simulink model "FSAE_UnifiedControl_ClosedLoop"  (R2026a)
settings: Solver=ode45  StopTime=10  MaxStep=0.01
model workspace (MAT data in the model file):
  PathTrackingAntiWindupGain = 0.5
  PathTrackingBrakePressurePerAcceleration = 10000
  PathTrackingControlSampleTime = 0.01
  PathTrackingCrossTrackGain = 2
  PathTrackingEnvironment.RoadGripScale = [1; 1; 1; 1]
  PathTrackingEnvironment.RoadMuLimit = [Inf; Inf; Inf; Inf]
  PathTrackingEnvironment.RoadGrade = 0
  PathTrackingEnvironment.RoadBank = 0
  PathTrackingEnvironment.RoadHeight = [0; 0; 0; 0]
  PathTrackingEnvironment.AirDensity = 1.225
  PathTrackingEnvironment.WindVelocityGlobal = [0; 0; 0]
  PathTrackingEnvironment.AmbientTemperature = 25
  PathTrackingEnvironment.Gravity = 9.80665
  PathTrackingEnvironment.EnableRoadDisturbance = 0
  PathTrackingEnvironment.EnvironmentValid = 1
  PathTrackingHeadingGain = 1.2
  PathTrackingLookaheadTime = 0.1
  PathTrackingMaximumAcceleration = 8
  PathTrackingMaximumDeceleration = 8
  PathTrackingMaximumSteeringAngle = 0.5
  PathTrackingMaximumSteeringRate = 4
  PathTrackingMinLookahead = 0.5
  PathTrackingMinimumSteeringSpeed = 1
  PathTrackingProjectionSearchWindow = 200
  PathTrackingSpeedKi = 0.25
  PathTrackingSpeedKp = 0.8
  PathTrackingSteeringWheelRatio = 1
  PathTrackingTrackData.SampleCount = 150
  PathTrackingTrackData.SampleDistance = 0.503355704698
  PathTrackingTrackData.TrackLength = 75
  PathTrackingTrackData.IsClosed = 0
  PathTrackingTrackData.ReferencePathValid = 0
  PathTrackingTrackData.ReferenceSampleDistance = 0.503355704698
  PathTrackingTrackData.X = [0 0.503355704698 1.0067114094 1.51006711409 2.01342281879 2.51677852349 3.02013422819 3.52348993289 4.02684563758 4.53020134228 5.03355704698 5.53691275168 ... (4096 elements, 4096x1)]
  PathTrackingTrackData.Y = [0 0 0 0 0 0 0 0 0 0 0 0 ... (4096 elements, 4096x1)]
  PathTrackingTrackData.Heading = [0 0 0 0 0 0 0 0 0 0 0 0 ... (4096 elements, 4096x1)]
  PathTrackingTrackData.Curvature = [0 0 0 0 0 0 0 0 0 0 0 0 ... (4096 elements, 4096x1)]
  PathTrackingTrackData.ReferenceX = [0 0.503355704698 1.0067114094 1.51006711409 2.01342281879 2.51677852349 3.02013422819 3.52348993289 4.02684563758 4.53020134228 5.03355704698 5.53691275168 ... (4096 elements, 4096x1)]
  PathTrackingTrackData.ReferenceY = [0 0 0 0 0 0 0 0 0 0 0 0 ... (4096 elements, 4096x1)]
  PathTrackingTrackData.ReferenceHeading = [0 0 0 0 0 0 0 0 0 0 0 0 ... (4096 elements, 4096x1)]
  PathTrackingTrackData.ReferenceCurvature = [0 0 0 0 0 0 0 0 0 0 0 0 ... (4096 elements, 4096x1)]
  PathTrackingTrackData.ReferenceEnvelopeClearance = [1.79769313486e+308 1.79769313486e+308 1.79769313486e+308 1.79769313486e+308 1.79769313486e+308 1.79769313486e+308 1.79769313486e+308 1.79769313486e+308 1.79769313486e+308 1.79769313486e+308 1.79769313486e+308 1.79769313486e+308 ... (4096 elements, 4096x1)]
  PathTrackingTrackData.ReferenceBoundaryCorrectionSign = [0 0 0 0 0 0 0 0 0 0 0 0 ... (4096 elements, 4096x1)]
  PathTrackingTrackData.ReferenceSpeed = [30 30 30 30 30 30 30 30 30 30 30 30 ... (4096 elements, 4096x1)]
  PathTrackingTrackData.LeftHalfWidth = [1.5 1.5 1.5 1.5 1.5 1.5 1.5 1.5 1.5 1.5 1.5 1.5 ... (4096 elements, 4096x1)]
  PathTrackingTrackData.RightHalfWidth = [1.5 1.5 1.5 1.5 1.5 1.5 1.5 1.5 1.5 1.5 1.5 1.5 ... (4096 elements, 4096x1)]
  PathTrackingWheelbase = 2
undefined symbols (not defined in the file): DefaultPowertrainStateBus, DefaultSensorBus
settings Model: DataDictionary=VehicleData.sldd  Creator=Xu Dingyi  LastModifiedBy=Xu Dingyi
settings SolverCC: ZeroCrossAlgorithm=Adaptive
settings DebuggingCC: AlgebraicLoopMsg=error  IgnoredZcDiagnostic=none  BusObjectLabelMismatch=error

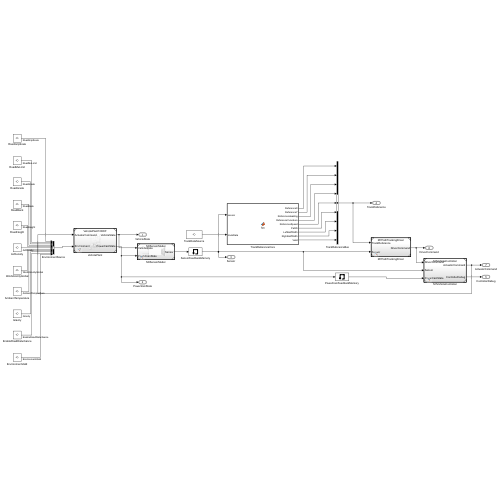
[thumbnail: Simulink's stored preview of the top-level diagram]
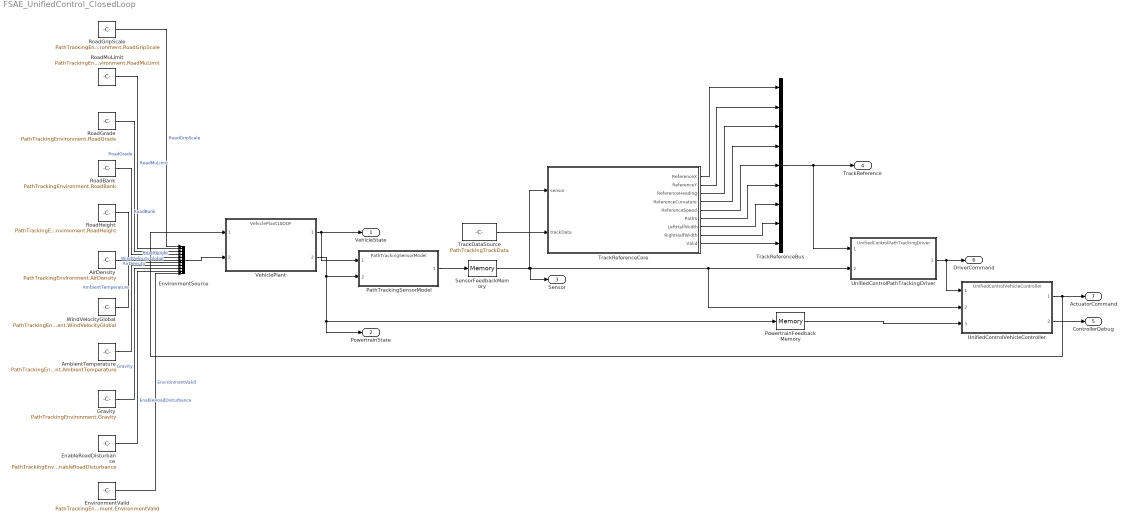
== system FSAE_UnifiedControl_ClosedLoop ==
  AirDensity : Constant  Value=PathTrackingEnvironment.AirDensity
  AmbientTemperature : Constant  Value=PathTrackingEnvironment.AmbientTemperature
  EnableRoadDisturbance : Constant  Value=PathTrackingEnvironment.EnableRoadDisturbance
  EnvironmentSource : BusCreator  Inputs=11  OutDataTypeStr=Bus: EnvironmentBus
  EnvironmentValid : Constant  Value=PathTrackingEnvironment.EnvironmentValid
  Gravity : Constant  Value=PathTrackingEnvironment.Gravity
  PathTrackingSensorModel : ModelReference  ModelNameDialog=PathTrackingSensorModel  SimulationMode=Normal  ModelReferenceVersion=1.2
  PowertrainFeedbackMemory : Memory  InitialCondition=DefaultPowertrainStateBus
  RoadBank : Constant  Value=PathTrackingEnvironment.RoadBank
  RoadGrade : Constant  Value=PathTrackingEnvironment.RoadGrade
  RoadGripScale : Constant  Value=PathTrackingEnvironment.RoadGripScale
  RoadHeight : Constant  Value=PathTrackingEnvironment.RoadHeight
  RoadMuLimit : Constant  Value=PathTrackingEnvironment.RoadMuLimit
  SensorFeedbackMemory : Memory  InitialCondition=DefaultSensorBus
  TrackDataSource : Constant  Value=PathTrackingTrackData  OutDataTypeStr=Bus: PathTrackingTrackDataBus
  TrackReferenceBus : BusCreator  Inputs=9  OutDataTypeStr=Bus: TrackReferenceBus
  TrackReferenceCore : MATLAB Function  TreatAsAtomicUnit=on
  UnifiedControlPathTrackingDriver : ModelReference  ModelNameDialog=UnifiedControlPathTrackingDriver  SimulationMode=Normal  ModelReferenceVersion=1.2
  UnifiedControlVehicleController : ModelReference  ModelNameDialog=UnifiedControlVehicleController  SimulationMode=Normal  ModelReferenceVersion=1.2
  VehiclePlant : ModelReference  ModelNameDialog=VehiclePlant10DOF  SimulationMode=Normal  ModelReferenceVersion=1.22
  WindVelocityGlobal : Constant  Value=PathTrackingEnvironment.WindVelocityGlobal
  VehicleState : Outport  OutDataTypeStr=Bus: VehicleStateBus
  PowertrainState : Outport  Port=2  OutDataTypeStr=Bus: PowertrainStateBus
  Sensor : Outport  Port=3  OutDataTypeStr=Bus: SensorBus
  TrackReference : Outport  Port=4  OutDataTypeStr=Bus: TrackReferenceBus
  ControllerDebug : Outport  Port=5  OutDataTypeStr=Bus: ControllerDebugBus
  DriverCommand : Outport  Port=6  OutDataTypeStr=Bus: DriverCommandBus
  ActuatorCommand : Outport  Port=7  OutDataTypeStr=Bus: ActuatorCommandBus
  wires:
  PathTrackingSensorModel/1 -> SensorFeedbackMemory/1
  SensorFeedbackMemory/1 -> UnifiedControlPathTrackingDriver/2, UnifiedControlVehicleController/2, Sensor/1, TrackReferenceCore/1(sensor)
  TrackDataSource/1 -> TrackReferenceCore/2(trackData)
  VehiclePlant/1 -> PathTrackingSensorModel/1, VehicleState/1
  VehiclePlant/2 -> PowertrainState/1, PowertrainFeedbackMemory/1, PathTrackingSensorModel/2
  TrackReferenceCore/1(ReferenceX) -> TrackReferenceBus/1
  TrackReferenceCore/2(ReferenceY) -> TrackReferenceBus/2
  TrackReferenceCore/3(ReferenceHeading) -> TrackReferenceBus/3
  TrackReferenceCore/4(ReferenceCurvature) -> TrackReferenceBus/4
  TrackReferenceCore/5(ReferenceSpeed) -> TrackReferenceBus/5
  TrackReferenceCore/6(PathS) -> TrackReferenceBus/6
  TrackReferenceCore/7(LeftHalfWidth) -> TrackReferenceBus/7
  UnifiedControlPathTrackingDriver/1 -> UnifiedControlVehicleController/1, DriverCommand/1
  TrackReferenceCore/8(RightHalfWidth) -> TrackReferenceBus/8
  TrackReferenceCore/9(Valid) -> TrackReferenceBus/9
  TrackReferenceBus/1 -> UnifiedControlPathTrackingDriver/1, TrackReference/1
  PowertrainFeedbackMemory/1 -> UnifiedControlVehicleController/3
  UnifiedControlVehicleController/1 -> VehiclePlant/1, ActuatorCommand/1
  UnifiedControlVehicleController/2 -> ControllerDebug/1
  EnvironmentSource/1 -> VehiclePlant/2
  RoadGripScale/1 -> EnvironmentSource/1  "RoadGripScale"
  RoadMuLimit/1 -> EnvironmentSource/2  "RoadMuLimit"
  RoadGrade/1 -> EnvironmentSource/3  "RoadGrade"
  RoadBank/1 -> EnvironmentSource/4  "RoadBank"
  RoadHeight/1 -> EnvironmentSource/5  "RoadHeight"
  AirDensity/1 -> EnvironmentSource/6  "AirDensity"
  WindVelocityGlobal/1 -> EnvironmentSource/7  "WindVelocityGlobal"
  AmbientTemperature/1 -> EnvironmentSource/8  "AmbientTemperature"
  Gravity/1 -> EnvironmentSource/9  "Gravity"
  EnableRoadDisturbance/1 -> EnvironmentSource/10  "EnableRoadDisturbance"
  EnvironmentValid/1 -> EnvironmentSource/11  "EnvironmentValid"

== matlab function FSAE_UnifiedControl_ClosedLoop/TrackReferenceCore ==
  data: sensor input; ReferenceX output; trackData input; ReferenceY output; ReferenceHeading output; ReferenceCurvature output; ReferenceSpeed output; PathS output; LeftHalfWidth output; RightHalfWidth output; Valid output; PathTrackingProjectionSearchWindow parameter; PathTrackingMinLookahead parameter; PathTrackingLookaheadTime parameter
function [ReferenceX, ReferenceY, ReferenceHeading, ReferenceCurvature, ...
    ReferenceSpeed, PathS, LeftHalfWidth, RightHalfWidth, Valid] = ...
    fcn(sensor, trackData, PathTrackingProjectionSearchWindow, PathTrackingMinLookahead, PathTrackingLookaheadTime)
%FSAEPathTrackingTRACKREFERENCECORE Code-generation-safe projection and look-ahead.

persistent previousIndex
if isempty(previousIndex)
    previousIndex = 1;
end

sampleCount = double(trackData.SampleCount);
Valid = false;
ReferenceX = 0;
ReferenceY = 0;
ReferenceHeading = 0;
ReferenceCurvature = 0;
ReferenceSpeed = 0;
PathS = 0;
LeftHalfWidth = 0;
RightHalfWidth = 0;
if sampleCount < 2 || ~sensor.PoseValid
    return
end

if previousIndex < 1 || previousIndex > sampleCount
    previousIndex = 1;
end
window = min(PathTrackingProjectionSearchWindow, floor(sampleCount / 2));
bestIndex = previousIndex;
bestDistance = realmax;
for offset = -window:window
    if trackData.IsClosed
        candidate = mod(previousIndex - 1 + offset, sampleCount) + 1;
    else
        candidate = min(sampleCount, max(1, previousIndex + offset));
    end
    distance = (trackData.X(candidate) - sensor.PositionX)^2 + ...
        (trackData.Y(candidate) - sensor.PositionY)^2;
    if distance < bestDistance
        bestDistance = distance;
        bestIndex = candidate;
    end
end
previousIndex = bestIndex;

currentS = (bestIndex - 1) * trackData.SampleDistance;
lookAhead = max(PathTrackingMinLookahead, ...
    abs(sensor.LongitudinalSpeed) * PathTrackingLookaheadTime);
if trackData.IsClosed
    targetS = mod(currentS + lookAhead, trackData.TrackLength);
    targetIndex = mod(round(targetS / trackData.SampleDistance), sampleCount) + 1;
else
    targetS = min(trackData.TrackLength, currentS + lookAhead);
    targetIndex = min(sampleCount, round(targetS / trackData.SampleDistance) + 1);
end

ReferenceX = trackData.X(targetIndex);
ReferenceY = trackData.Y(targetIndex);
ReferenceHeading = trackData.Heading(targetIndex);
ReferenceCurvature = trackData.Curvature(targetIndex);
ReferenceSpeed = trackData.ReferenceSpeed(targetIndex);
PathS = targetS;
LeftHalfWidth = trackData.LeftHalfWidth(targetIndex);
RightHalfWidth = trackData.RightHalfWidth(targetIndex);
Valid = true;
end
